simulink model "navigator_test"  (R2013b)
settings: Solver=ode45  StartTime=0.0  StopTime=10.0  RelTol=1e-3
undefined symbols (not defined in the file): Earth, WGS84
libraries: aerolibtransform2 x3, simulink_extras x2
settings Model: Creator=Gianluca Rossetti  LastModifiedBy=Gianluca Rossetti

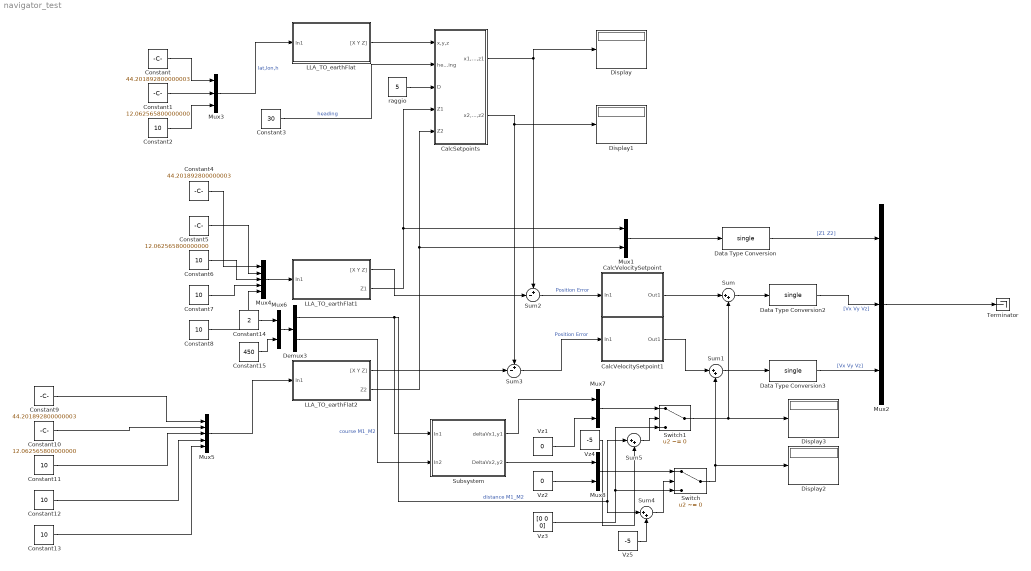
== system navigator_test ==
  CalcSetpoints : Subsystem
  CalcVelocitySetpoint : Subsystem
  CalcVelocitySetpoint1 : Subsystem
  Constant : Constant  Value=44.201892800000003
  Constant1 : Constant  Value=12.062565800000000
  Constant10 : Constant  Value=12.062565800000000
  Constant{2,6..8,11..13} (7 alike) : Constant  Value=10
  Constant14 : Constant  Value=2
  Constant15 : Constant  Value=450
  Constant3 : Constant  Value=30
  Constant4 : Constant  Value=44.201892800000003
  Constant5 : Constant  Value=12.062565800000000
  Constant9 : Constant  Value=44.201892800000003
  Data Type Conversion : DataTypeConversion  OutDataTypeStr=single
  Data Type Conversion2 : DataTypeConversion  OutDataTypeStr=single
  Data Type Conversion3 : DataTypeConversion  OutDataTypeStr=single
  Demux3 : Demux  Outputs=2
  Display{,1..3} (4 alike) : Display
  LLA_TO_earthFlat : Subsystem
  LLA_TO_earthFlat1 : Subsystem
  LLA_TO_earthFlat2 : Subsystem
  Mux1 : Mux  Inputs=[1 1]
  Mux2 : Mux  Inputs=[2 3 3]
  Mux3 : Mux  Inputs=[1 1 1]
  Mux4 : Mux  Inputs=[1 1 1 1 1]
  Mux5 : Mux  Inputs=[1 1 1 1 1]
  Mux6 : Mux  Inputs=[1 1]
  Mux7 : Mux  Inputs=[2 1]
  Mux8 : Mux  Inputs=[2 1]
  Subsystem : Subsystem
  Sum{,1,4..5} (4 alike) : Sum  Inputs=|++
  Sum2 : Sum  Inputs=+-|
  Sum3 : Sum  Inputs=+-|
  Switch : Switch  Criteria=u2 ~= 0  Threshold=5
  Switch1 : Switch  Criteria=u2 ~= 0  Threshold=5
  Terminator : Terminator
  Vz1 : Constant  Value=0
  Vz2 : Constant  Value=0
  Vz3 : Constant  Value=[0 0 0]
  Vz4 : Constant  Value=-5
  Vz5 : Constant  Value=-5
  raggio : Constant  Value=5
  wires:
  Data Type Conversion/1 -> Mux2/1  "[Z1 Z2]"
  Mux2/1 -> Terminator/1
  LLA_TO_earthFlat1/1("[X Y Z]") -> Sum2/2
  Data Type Conversion2/1 -> Mux2/2  "[Vx Vy Vz]"
  Sum2/1 -> CalcVelocitySetpoint/1(In1)  "Position Error"
  CalcVelocitySetpoint/1(Out1) -> Sum/1
  LLA_TO_earthFlat2/1("[X Y Z]") -> Sum3/2
  Sum3/1 -> CalcVelocitySetpoint1/1(In1)  "Position Error"
  CalcVelocitySetpoint1/1(Out1) -> Sum1/1
  Data Type Conversion3/1 -> Mux2/3  "[Vx Vy Vz]"
  Mux3/1 -> LLA_TO_earthFlat/1(In1)  "lat,lon,h"
  LLA_TO_earthFlat/1("[X Y Z]") -> CalcSetpoints/1(x,y,z)
  Constant3/1 -> CalcSetpoints/2(heading)  "heading"
  CalcSetpoints/1(x1,y1,z1) -> Display/1, Sum2/1
  CalcSetpoints/2(x2,y2,z2) -> Display1/1, Sum3/1
  raggio/1 -> CalcSetpoints/3(D)
  LLA_TO_earthFlat1/2(Z1) -> CalcSetpoints/4(Z1), Mux1/1
  LLA_TO_earthFlat2/2(Z2) -> CalcSetpoints/5(Z2), Mux1/2
  Demux3/1 -> Sum5/1, Sum4/1, Subsystem/1(In1)  "distance M1_M2"
  Sum/1 -> Data Type Conversion2/1
  Sum1/1 -> Data Type Conversion3/1
  Subsystem/2(DeltaVx2,y2) -> Mux8/1
  Mux1/1 -> Data Type Conversion/1
  Constant/1 -> Mux3/1
  Constant2/1 -> Mux3/3
  Constant1/1 -> Mux3/2
  Constant7/1 -> Mux4/4
  Constant6/1 -> Mux4/3
  Constant8/1 -> Mux4/5
  Constant5/1 -> Mux4/2
  Constant4/1 -> Mux4/1
  Mux4/1 -> LLA_TO_earthFlat1/1(In1)
  Constant12/1 -> Mux5/4
  Constant11/1 -> Mux5/3
  Constant13/1 -> Mux5/5
  Constant10/1 -> Mux5/2
  Constant9/1 -> Mux5/1
  Mux5/1 -> LLA_TO_earthFlat2/1(In1)
  Mux6/1 -> Demux3/1
  Constant14/1 -> Mux6/1
  Constant15/1 -> Mux6/2
  Demux3/2 -> Subsystem/2(In2)  "course M1_M2"
  Vz2/1 -> Mux8/2
  Mux8/1 -> Switch/1
  Switch/1 -> Sum1/2, Display2/1
  Vz3/1 -> Switch1/3, Switch/3
  Subsystem/1(deltaVx1,y1) -> Mux7/1
  Vz1/1 -> Mux7/2
  Mux7/1 -> Switch1/1
  Switch1/1 -> Sum/2, Display3/1
  Sum4/1 -> Switch/2
  Sum5/1 -> Switch1/2
  Vz5/1 -> Sum4/2
  Vz4/1 -> Sum5/2

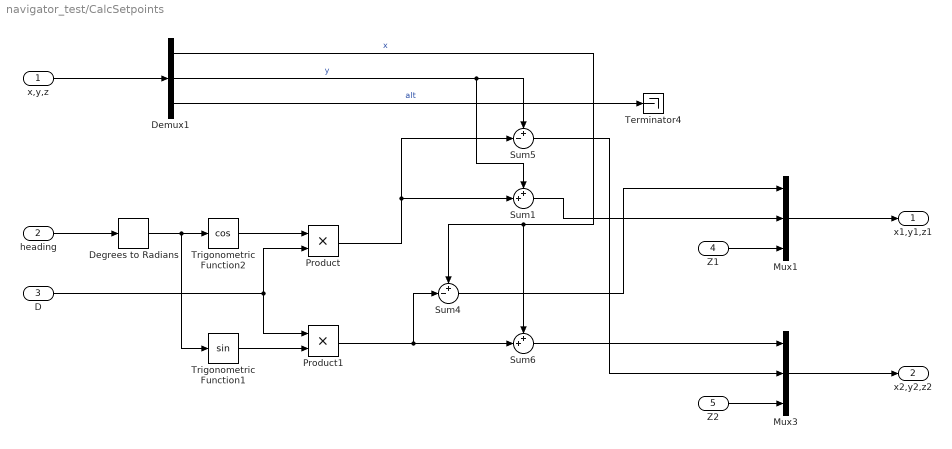
== system navigator_test/CalcSetpoints ==
  x,y,z : Inport
  heading : Inport  Port=2
  D : Inport  Port=3
  Z1 : Inport  Port=4
  Z2 : Inport  Port=5
  Degrees to Radians : simulink_extras/Transformations/Degrees to Radians
  Demux1 : Demux  Outputs=[1 1 1]
  Mux1 : Mux  Inputs=[1 1 1]
  Mux3 : Mux  Inputs=[1 1 1]
  Product : Product
  Product1 : Product
  Sum1 : Sum  Inputs=++|
  Sum4 : Sum  Inputs=+-|
  Sum5 : Sum  Inputs=+-|
  Sum6 : Sum  Inputs=++|
  Terminator4 : Terminator
  Trigonometric Function1 : Trigonometry
  Trigonometric Function2 : Trigonometry  Operator=cos
  x1,y1,z1 : Outport
  x2,y2,z2 : Outport  Port=2
  wires:
  Sum5/1 -> Mux3/2
  Sum6/1 -> Mux3/1
  Mux3/1 -> x2,y2,z2/1
  Demux1/1 -> Sum4/1, Sum6/1  "x"
  Mux1/1 -> x1,y1,z1/1
  Sum4/1 -> Mux1/1
  Product1/1 -> Sum6/2, Sum4/2
  heading/1 -> Degrees to Radians/1
  Demux1/2 -> Sum5/1, Sum1/1  "y"
  Sum1/1 -> Mux1/2
  Demux1/3 -> Terminator4/1  "alt"
  Product/1 -> Sum5/2, Sum1/2
  D/1 -> Product1/1, Product/2
  x,y,z/1 -> Demux1/1
  Degrees to Radians/1 -> Trigonometric Function1/1, Trigonometric Function2/1
  Trigonometric Function2/1 -> Product/1
  Trigonometric Function1/1 -> Product1/2
  Z2/1 -> Mux3/3
  Z1/1 -> Mux1/3

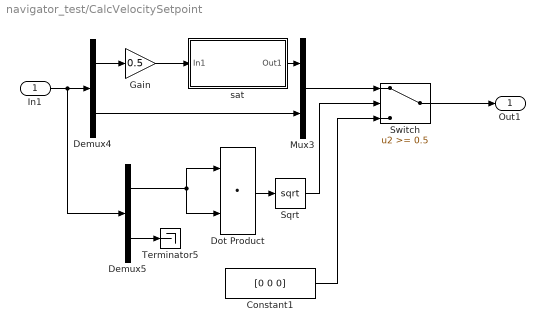
== system navigator_test/CalcVelocitySetpoint ==
  In1 : Inport
  Constant1 : Constant  Value=[0 0 0]
  Demux4 : Demux  Outputs=[2 1]
  Demux5 : Demux  Outputs=[2 1]
  Dot Product : DotProduct  InputSameDT=on  OutDataTypeStr=Inherit: Inherit via internal rule
  Gain : Gain  Gain=0.5
  Mux3 : Mux  Inputs=[2 1]
  Sqrt : Sqrt  SaturateOnIntegerOverflow=on
  Switch : Switch  Threshold=0.5
  Terminator5 : Terminator
  "sat " : Subsystem  mask{k_sat=5}
      mask prompts: k_sat "Saturatore"
  Out1 : Outport
  wires:
  In1/1 -> Demux4/1, Demux5/1
  Demux4/1 -> Gain/1
  "sat "/1(Out1) -> Mux3/1
  Demux4/2 -> Mux3/2
  Demux5/1 -> Dot Product/1, Dot Product/2
  Dot Product/1 -> Sqrt/1
  Demux5/2 -> Terminator5/1
  Sqrt/1 -> Switch/2
  Mux3/1 -> Switch/1
  Constant1/1 -> Switch/3
  Switch/1 -> Out1/1
  Gain/1 -> "sat "/1(In1)

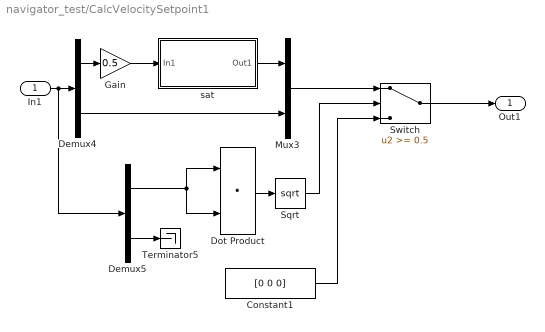
== system navigator_test/CalcVelocitySetpoint1 ==
  In1 : Inport
  Constant1 : Constant  Value=[0 0 0]
  Demux4 : Demux  Outputs=[2 1]
  Demux5 : Demux  Outputs=[2 1]
  Dot Product : DotProduct  InputSameDT=on  OutDataTypeStr=Inherit: Inherit via internal rule
  Gain : Gain  Gain=0.5
  Mux3 : Mux  Inputs=[2 1]
  Sqrt : Sqrt  SaturateOnIntegerOverflow=on
  Switch : Switch  Threshold=0.5
  Terminator5 : Terminator
  "sat " : Subsystem  mask{k_sat=5}
      mask prompts: k_sat "Saturatore"
  Out1 : Outport
  wires:
  Switch/1 -> Out1/1
  Constant1/1 -> Switch/3
  Mux3/1 -> Switch/1
  Sqrt/1 -> Switch/2
  Demux5/2 -> Terminator5/1
  Dot Product/1 -> Sqrt/1
  Demux5/1 -> Dot Product/2, Dot Product/1
  Demux4/2 -> Mux3/2
  "sat "/1(Out1) -> Mux3/1
  Demux4/1 -> Gain/1
  In1/1 -> Demux4/1, Demux5/1
  Gain/1 -> "sat "/1(In1)

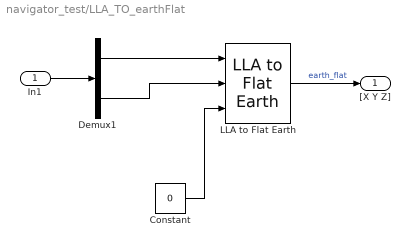
== system navigator_test/LLA_TO_earthFlat ==
  In1 : Inport
  Constant : Constant  Value=0  OutDataTypeStr=single
  Demux1 : Demux  Outputs=[2 1]
  LLA to Flat Earth : aerolibtransform2/LLA to Flat Earth  units=Metric (MKS)  ptype=Earth (WGS84)  F=1/298.257223563  R=6378137  LL0="[44.201892800000003  12.062565800000000]"  psi=0
  "[X Y Z]" : Outport
  wires:
  Constant/1 -> LLA to Flat Earth/3
  Demux1/1 -> LLA to Flat Earth/1
  LLA to Flat Earth/1 -> "[X Y Z]"/1  "earth_flat"
  Demux1/2 -> LLA to Flat Earth/2
  In1/1 -> Demux1/1

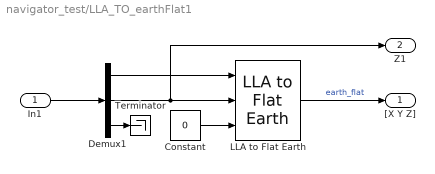
== system navigator_test/LLA_TO_earthFlat1 ==
  In1 : Inport
  Constant : Constant  Value=0  OutDataTypeStr=single
  Demux1 : Demux  Outputs=[2 1 2]
  LLA to Flat Earth : aerolibtransform2/LLA to Flat Earth  units=Metric (MKS)  ptype=Earth (WGS84)  F=1/298.257223563  R=6378137  LL0="[44.201892800000003  12.062565800000000]"  psi=0
  Terminator : Terminator
  "[X Y Z]" : Outport
  Z1 : Outport  Port=2
  wires:
  Demux1/3 -> Terminator/1
  In1/1 -> Demux1/1
  Demux1/2 -> Z1/1, LLA to Flat Earth/2
  LLA to Flat Earth/1 -> "[X Y Z]"/1  "earth_flat"
  Demux1/1 -> LLA to Flat Earth/1
  Constant/1 -> LLA to Flat Earth/3

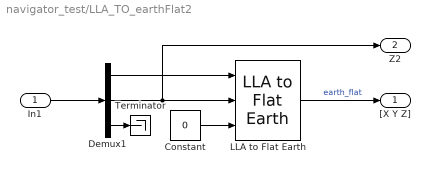
== system navigator_test/LLA_TO_earthFlat2 ==
  In1 : Inport
  Constant : Constant  Value=0  OutDataTypeStr=single
  Demux1 : Demux  Outputs=[2 1 2]
  LLA to Flat Earth : aerolibtransform2/LLA to Flat Earth  units=Metric (MKS)  ptype=Earth (WGS84)  F=1/298.257223563  R=6378137  LL0="[44.201892800000003  12.062565800000000]"  psi=0
  Terminator : Terminator
  "[X Y Z]" : Outport
  Z2 : Outport  Port=2
  wires:
  Constant/1 -> LLA to Flat Earth/3
  Demux1/1 -> LLA to Flat Earth/1
  LLA to Flat Earth/1 -> "[X Y Z]"/1  "earth_flat"
  Demux1/2 -> Z2/1, LLA to Flat Earth/2
  In1/1 -> Demux1/1
  Demux1/3 -> Terminator/1

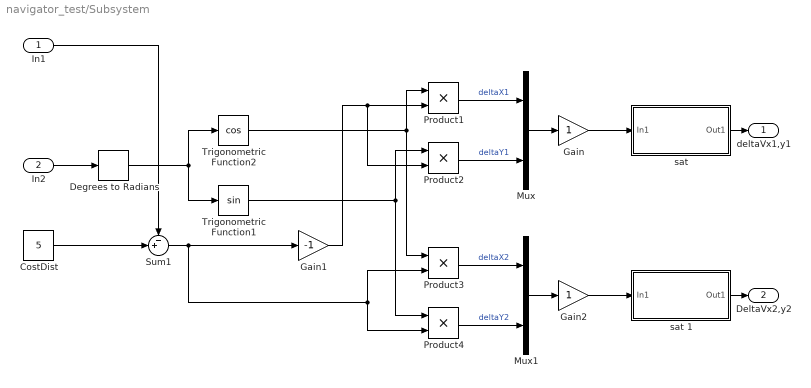
== system navigator_test/Subsystem ==
  In1 : Inport
  In2 : Inport  Port=2
  CostDist : Constant  Value=5
  Degrees to Radians : simulink_extras/Transformations/Degrees to Radians
  Gain : Gain
  Gain1 : Gain  Gain=-1
  Gain2 : Gain
  Mux : Mux  Inputs=2
  Mux1 : Mux  Inputs=2
  Product{1..4} (4 alike) : Product
  Sum1 : Sum  Inputs=-+|
  Trigonometric Function1 : Trigonometry
  Trigonometric Function2 : Trigonometry  Operator=cos
  "sat " : Subsystem  mask{k_sat=5}
      mask prompts: k_sat "Saturatore"
  sat 1 : Subsystem  mask{k_sat=5}
      mask prompts: k_sat "Saturatore"
  deltaVx1,y1 : Outport
  DeltaVx2,y2 : Outport  Port=2
  wires:
  Product2/1 -> Mux/2  "deltaY1"
  Product1/1 -> Mux/1  "deltaX1"
  Sum1/1 -> Product3/2, Product4/2, Gain1/1
  Gain/1 -> "sat "/1(In1)
  Product3/1 -> Mux1/1  "deltaX2"
  sat 1/1(Out1) -> DeltaVx2,y2/1
  Gain1/1 -> Product2/2, Product1/2
  Mux/1 -> Gain/1
  Trigonometric Function2/1 -> Product1/1, Product3/1
  Degrees to Radians/1 -> Trigonometric Function2/1, Trigonometric Function1/1
  In1/1 -> Sum1/1
  "sat "/1(Out1) -> deltaVx1,y1/1
  Gain2/1 -> sat 1/1(In1)
  In2/1 -> Degrees to Radians/1
  Mux1/1 -> Gain2/1
  Trigonometric Function1/1 -> Product2/1, Product4/1
  Product4/1 -> Mux1/2  "deltaY2"
  CostDist/1 -> Sum1/2

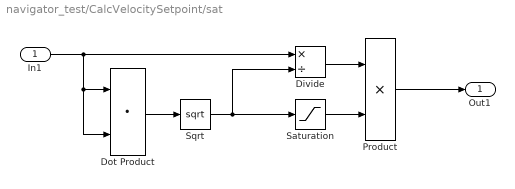
== system navigator_test/CalcVelocitySetpoint/sat  ==
  In1 : Inport
  Divide : Product  Inputs=*/
  Dot Product : DotProduct  InputSameDT=on  OutDataTypeStr=Inherit: Inherit via internal rule
  Product : Product
  Saturation : Saturate  UpperLimit=k_sat  LowerLimit=0
  Sqrt : Sqrt  SaturateOnIntegerOverflow=on
  Out1 : Outport
  wires:
  Divide/1 -> Product/1
  Product/1 -> Out1/1
  Sqrt/1 -> Divide/2, Saturation/1
  In1/1 -> Divide/1, Dot Product/1, Dot Product/2
  Dot Product/1 -> Sqrt/1
  Saturation/1 -> Product/2

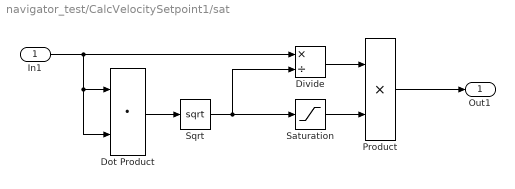
== system navigator_test/CalcVelocitySetpoint1/sat  ==
  In1 : Inport
  Divide : Product  Inputs=*/
  Dot Product : DotProduct  InputSameDT=on  OutDataTypeStr=Inherit: Inherit via internal rule
  Product : Product
  Saturation : Saturate  UpperLimit=k_sat  LowerLimit=0
  Sqrt : Sqrt  SaturateOnIntegerOverflow=on
  Out1 : Outport
  wires:
  Saturation/1 -> Product/2
  Dot Product/1 -> Sqrt/1
  In1/1 -> Dot Product/2, Dot Product/1, Divide/1
  Sqrt/1 -> Saturation/1, Divide/2
  Product/1 -> Out1/1
  Divide/1 -> Product/1

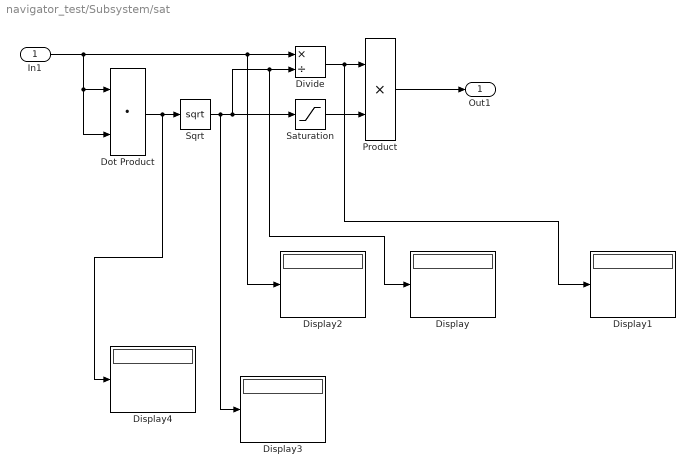
== system navigator_test/Subsystem/sat  ==
  In1 : Inport
  Display{,1..4} (5 alike) : Display
  Divide : Product  Inputs=*/
  Dot Product : DotProduct  InputSameDT=on  OutDataTypeStr=Inherit: Inherit via internal rule
  Product : Product
  Saturation : Saturate  UpperLimit=k_sat  LowerLimit=0
  Sqrt : Sqrt  SaturateOnIntegerOverflow=on
  Out1 : Outport
  wires:
  Divide/1 -> Display1/1, Product/1
  Sqrt/1 -> Display3/1, Display/1, Divide/2, Saturation/1
  In1/1 -> Display2/1, Divide/1, Dot Product/1, Dot Product/2
  Saturation/1 -> Product/2
  Product/1 -> Out1/1
  Dot Product/1 -> Display4/1, Sqrt/1

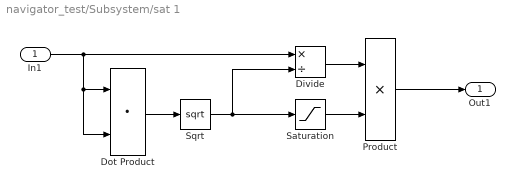
== system navigator_test/Subsystem/sat 1 ==
  In1 : Inport
  Divide : Product  Inputs=*/
  Dot Product : DotProduct  InputSameDT=on  OutDataTypeStr=Inherit: Inherit via internal rule
  Product : Product
  Saturation : Saturate  UpperLimit=k_sat  LowerLimit=0
  Sqrt : Sqrt  SaturateOnIntegerOverflow=on
  Out1 : Outport
  wires:
  Saturation/1 -> Product/2
  Dot Product/1 -> Sqrt/1
  In1/1 -> Dot Product/2, Dot Product/1, Divide/1
  Sqrt/1 -> Saturation/1, Divide/2
  Product/1 -> Out1/1
  Divide/1 -> Product/1
